simulink model "QPSK_synch_baseband"  (R2014b)
settings: Solver=VariableStepDiscrete  StartTime=0.0  StopTime=100000/fs  RelTol=1e-3
PreLoadFcn:
  | %%%%%%%%%%%%%%%%%%%%%%%%%%%%%%%%%%%%%%%%%%%%%%%%%%%%%%%%%%%%%%%%%%%%%%%%%%%
  | % check to see if Simulink library folder is missing from the MATLAB path %
  | %%%%%%%%%%%%%%%%%%%%%%%%%%%%%%%%%%%%%%%%%%%%%%%%%%%%%%%%%%%%%%%%%%%%%%%%%%%
  | if isempty(strfind(path, 'rtlsdr_book_library'))
  | 
  |     % create error window
  |     fig_error = figure(...
  |         'Name', 'Error: RTL-SDR Book Library',...
  |         'Toolbar','none',...
  |         'MenuBar','none',...
  |         'NumberTitle','off',...
  |         'Resize','off',...
  |         'WindowStyle','modal');
  |     fig_error.Position(3) = 600;
  |     fig_error.Position(4) = 150;
  |     fig_axes = axes(...
  |         'Parent',fig_error,...
  |         'Position',[0,0,1,1],...
  |         'visible','off');
  |     % error message
  |     t_title = text(.05,.8,...
  |         'MISSING DIRECTORIES',...
  |         'FontSize',11.5);
  |     t_body = text(.075,.6,...
  |         [{'Simulink cannot find the  \it{<root>}\rm / \it{rtlsdr\_book\_library}\rm  folder in the \it{MATLAB Path}\rm.'},...
  |         {'Please set the MATLAB path following the instructions given in Exercise 2.4.'}],...
  |         'FontSize',10.5);
  |     % buttons
  |     btn_path = uicontrol(...
  |         'Parent',fig_error,...
  |         'String','Set Path Now',...
  |         'FontSize',10,...
  |         'Callback', 'pathtool; close(fig_error);',...
  |         'Position', [fig_error.Position(3)/2-210, 30, 200, 30]);
  |     btn_abort = uicontrol(...
  |         'Parent',fig_error,...
  |         'String','No thanks',...
  |         'FontSize',10,...
  |         'Callback', 'close(fig_error); abort=1;',...
  |         'Position', [fig_error.Position(3)/2+10, 30, 200, 30]);
  | 
  |     % pause to allow user to interact with error box
  |     uiwait(fig_error);
  | 
  |     % abort simulation
  |     try
  |         if abort==1
  |             set_param(gcs, 'SimulationCommand', 'stop');
  |         end
  |     end
  | 
  |     % if user has set path, allow diagram to be updated
  |     if ~exist('abort','var')
  |         % create error window
  |         fig_update = figure(...
  |             'Name', 'Update Diagram',...
  |             'Toolbar','none',...
  |             'MenuBar','none',...
  |             'NumberTitle','off',...
  |             'Resize','off');
  |         fig_update.Position(3) = 400;
  |         fig_update.Position(4) = 120;
  |         fig_axes = axes(...
  |             'Parent',fig_update,...
  |             'Position',[0,0,1,1],...
  |             'visible','off');
  |         % instruction message
  |         t_body = text(.075,.7,...
  |             'Once you have set the path, update the block diagram',...
  |             'FontSize',10.5);
  |         % button
  |         btn_update = uicontrol(...
  |             'Parent',fig_update,...
  |             'String','Update Block Diagram',...
  |             'FontSize',10,...
  |             'Callback', 'set_param(gcs,''SimulationCommand'',''update''); close(gcf)',...
  |             'Position', [fig_update.Position(3)/2-100, 30, 200, 30]);
  |     end
  | 
  |     % clear error components
  |     clear('fig_error','fig_update','fig_axes','t_title','t_body','btn_path','btn_abort','btn_update','abort');
  | 
  | end
  | %%%%%%%%%%%%%%%%%%%%%%%%%%%%%%%%%%%%%%%%%%%%%%%%%%%%%%%%%%%%%%%%%%%%%%%%%%%
  | 
  | 
  | Rdata = 100e3;
  | Rsymbol = Rdata/2;
  | fs = 2.4e6;
  | MHz = fs/1e6;
  | interp = fs/Rsymbol;
  | fc = 600e3;
  | fe = 400;                   % frequency error
  | 
  | % ------- new section for synch loop design --------
  | 
  | T = 1/fs;    % sample period
  | Kp = 1;      % phase detector S-curve is linear
  | Bn = 25000;   % noise bandwidth in Hz
  | Ko = 1;      % gain of NCO (here just a direct conversion)
  | 
  | d = 0.707;  % damping ratio
  | 
  | % calculate the loop filter coefficients
  | K1 = (4*d*Bn*T)/(Ko*Kp*(d+1/(4*d)));
  | K2 = (4*(Bn*T)^2)/(Ko*Kp*(d+1/4*d)^2);
undefined symbols (not defined in the file): startfcn_constellation, startfcn_time_scope
libraries: commfilt2 x4, commrandsrc2 x1, rtlsdr_book_library x1, commdigbbndpm3 x1
CloseFcn:
  | closefcn_model;
Description:
  | Software, Simulation Examples and Design Exercises Licence Agreement
  | 
  | This license agreement refers to the simulation examples, design exercises and files,
  | and associated software MATLAB and Simulink resources that accompany the book:
  | 
  |      Title: Software Defined Radio using MATLAB & Simulink and the RTL-SDR
  |      Published by Strathclyde Academic Media, 2015
  |      Authored by Robert W. Stewart, Kenneth W. Barlee, Dale S.W. Atkinson,
  |      and Louise H. Crockett
  | 
  | and made available as a download from, www.desktopSDR.com or variously acquired
  | by other means such as via USB storage, cloud storage, disk or any other electronic
  | or optical or magnetic storage mechanism. These files and associated software may
  | be used subject to the terms of agreement of the conditions below:
  | 
  |     Copyright © 2015 Robert W. Stewart, Kenneth W. Barlee, Dale S.W. Atkinson,
  |     and Louise H. Crockett
  |     All rights reserved.
  | 
  | Redistribution and use in source and binary forms, with or without modification, are
  | permitted provided that the following conditions are met:
  | 
  |    1.  Redistributions of source code must retain the above copyright notice, this list of
  |         conditions and the following disclaimer.
  | 
  |    2.  Redistributions in binary form must reproduce the above copyright notice, this
  |         list of conditions and the following disclaimer in the documentation and/or other
  |         materials provided with the distribution.
  | 
  |    3.  Neither the name of the copyright holder nor the names of its contributors may
  |         be used to endorse or promote products derived from this software without
  |         specific prior written permission.
  | 
  |    4.  In all cases, the software is, and all modifications and derivatives of the
  |         software shall be, licensed to you solely for use in conjunction with The
  |         MathWorks, Inc. products and service offerings.
  | 
  | THIS SOFTWARE IS PROVIDED BY THE COPYRIGHT HOLDERS AND CONTRIBUTORS
  | "AS IS" AND ANY EXPRESS OR IMPLIED WARRANTIES, INCLUDING, BUT NOT LIMITED
  | TO, THE IMPLIED WARRANTIES OF MERCHANTABILITY AND FITNESS FOR A
  | PARTICULAR PURPOSE ARE DISCLAIMED. IN NO EVENT SHALL THE COPYRIGHT
  | HOLDER OR CONTRIBUTORS BE LIABLE FOR ANY DIRECT, INDIRECT, INCIDENTAL,
  | SPECIAL, EXEMPLARY, OR CONSEQUENTIAL DAMAGES (INCLUDING, BUT NOT
  | LIMITED TO, PROCUREMENT OF SUBSTITUTE GOODS OR SERVICES; LOSS OF USE,
  | DATA, OR PROFITS; OR BUSINESS INTERRUPTION) HOWEVER CAUSED AND ON ANY
  | THEORY OF LIABILITY, WHETHER IN CONTRACT, STRICT LIABILITY, OR TORT
  | (INCLUDING NEGLIGENCE OR OTHERWISE) ARISING IN ANY WAY OUT OF THE USE
  | OF THIS SOFTWARE, EVEN IF ADVISED OF THE POSSIBILITY OF SUCH DAMAGE.
  | 
  | 
  | Audio Tracks used in Simulations Examples and Design Exercises
  | 
  | The music and vocal files used within the Examples files and software within the book
  | were variously written, arranged, performed, recorded and produced by Garrey Rice,
  | Adam Struth, Jamie Struth, Iain Thistlethwaite and also Marshall Craigmyle who
  | collectively, and individually where appropriate, assert and retain all of their copyright,
  | performance and artistic rights. Permission to use and reproduce this music is
  | granted for all purposes associated with MATLAB and Simulink software and the
  | simulation examples and design exercises files that accompany this book. Requests to
  | use the music for any other purpose should be directed to: info@desktopSDR.com.
  | For information on music track names, full credits, and links to the musicians please
  | refer to www.desktopSDR.com/more/audio.
settings Model: Creator=desktopSDR Team  LastModifiedBy=desktopSDR Team
settings DataIOCC: LimitDataPoints=off  SaveOutput=off  SignalLogging=off  SaveTime=off
settings DebuggingCC: UnderspecifiedInitializationDetection=Classic  MergeDetectMultiDrivingBlocksExec=none

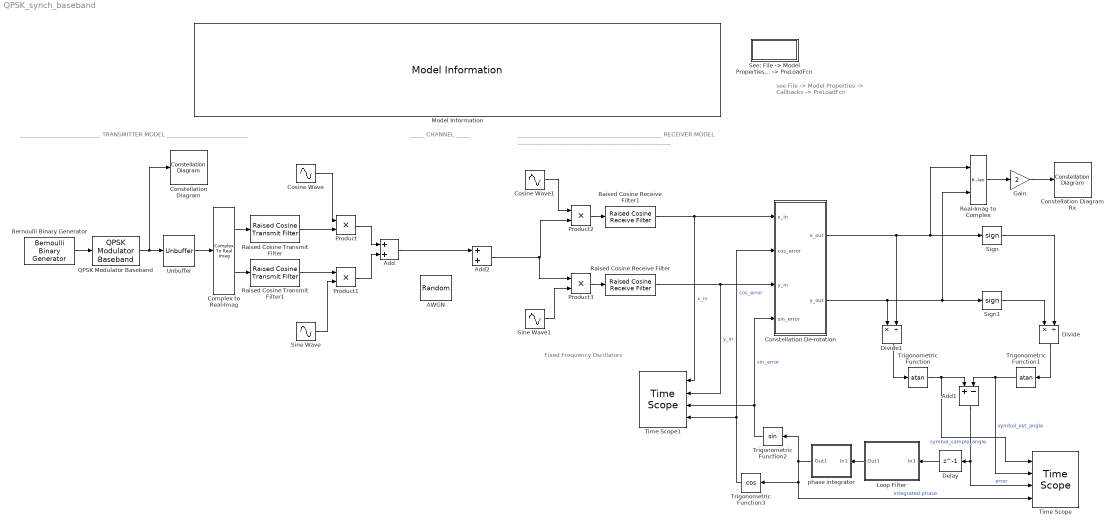
== system QPSK_synch_baseband ==
  note: Fixed Frequency
      | Oscillators
  note: ___________________________ TRANSMITTER MODEL ___________________________
  note: _____ CHANNEL _____
  note: ________________________________________________ RECEIVER MODEL ___________________________________________________
  note: see File -> Model Properties
      | -> Callbacks -> PreLoadFcn
  AWGN : RandomNumber  Variance=0.001  Seed=555  SampleTime=1/fs
  Add : Sum
  Add1 : Sum  Inputs=+-
  Add2 : Sum
  Bernoulli Binary Generator : commrandsrc2/Bernoulli Binary Generator  P=0.5  seed=61  Ts=1/Rdata  frameBased=on  sampPerFrame=2  orient=off  outDataType=double
  Complex to Real-Imag : ComplexToRealImag
  Constellation De-rotation : Subsystem
  Constellation Diagram : ConstellationDiagram  StartFcn=startfcn_constellation;
  Constellation Diagram Rx : ConstellationDiagram  StartFcn=startfcn_constellation;
  Cosine Wave : Sin  Frequency=(fc+fe)*2*pi  Phase=pi/2  SampleTime=1/fs
  Cosine Wave1 : Sin  Frequency=fc*2*pi  Phase=pi/2  SampleTime=1/fs
  Delay : Delay  DelayLength=1
  Divide : Product  Inputs=*/
  Divide1 : Product  Inputs=*/
  Gain : Gain  Gain=2
  Loop Filter : Subsystem
  Model Information : rtlsdr_book_library/Additional Tools/Model Information/Model Information
  Product{,1..3} (4 alike) : Product
  QPSK Modulator Baseband : commdigbbndpm3/QPSK Modulator Baseband  InType=Bit  Enc=Gray  Ph=pi/4  outDtype=double  outWordLen=16  outUDDataType=sfix(16)  outFracLenMode=Best precision  outFracLen=15
  Raised Cosine Receive Filter : commfilt2/Raised Cosine Receive Filter  filtType=Square root  N=interp  filtSpan=8  currentFiltSpan=8  D=(8)/2  R=0.25  sampMode=Mute  saveAsFlag=0  rateMode=Downsampling  downFactor=interp  downOffset=0  framing=Allow multirate processing  checkGain=Normalized  filterGain=1  checkCoeff=off  variableName=rcRxFilt  launchFVT=on  roundingMode=Floor  overflowMode=off
  Raised Cosine Receive Filter1 : commfilt2/Raised Cosine Receive Filter  filtType=Square root  N=interp  filtSpan=8  currentFiltSpan=8  D=(8)/2  R=0.25  sampMode=Mute  saveAsFlag=0  rateMode=Downsampling  downFactor=interp  downOffset=0  framing=Allow multirate processing  checkGain=Normalized  filterGain=1  checkCoeff=off  variableName=rcRxFilt1  launchFVT=on  roundingMode=Floor  overflowMode=off
  Raised Cosine Transmit Filter : commfilt2/Raised Cosine Transmit Filter  filtType=Square root  filtSpan=8  currentFiltSpan=8  D=(8)/2  R=0.25  sampMode=Mute  saveAsFlag=0  N=interp  framing=Allow multirate processing  checkGain=Normalized  filterGain=1  checkCoeff=off  variableName=rcTxFilt  launchFVT=on  roundingMode=Floor  overflowMode=off
  Raised Cosine Transmit Filter1 : commfilt2/Raised Cosine Transmit Filter  filtType=Square root  filtSpan=8  currentFiltSpan=8  D=(8)/2  R=0.25  sampMode=Mute  saveAsFlag=0  N=interp  framing=Allow multirate processing  checkGain=Normalized  filterGain=1  checkCoeff=off  variableName=rcTxFilt1  launchFVT=on  roundingMode=Floor  overflowMode=off
  Real-Imag to Complex : RealImagToComplex
  "See: File -> Model Properties -> Callbacks -> PreLoadFcn " : Subsystem
      mask Display:
      | MHz = evalin('base', 'MHz');
      | fprintf(['fs = ',num2str(MHz),' MHz']);
  Sign : Signum
  Sign1 : Signum
  Sine Wave : Sin  Frequency=(fc+fe)*2*pi  SampleTime=1/fs
  Sine Wave1 : Sin  Frequency=fc*2*pi  SampleTime=1/fs
  Time Scope : TimeScope  StartFcn=startfcn_time_scope;  DefaultConfigurationName=spbscopes.TimeScopeBlockCfg  NumInputPorts=4
  Time Scope1 : TimeScope  StartFcn=startfcn_time_scope;  DefaultConfigurationName=spbscopes.TimeScopeBlockCfg  NumInputPorts=4
  Trigonometric Function : Trigonometry  Operator=atan  OutputSignalType=real
  Trigonometric Function1 : Trigonometry  Operator=atan  OutputSignalType=real
  Trigonometric Function2 : Trigonometry
  Trigonometric Function3 : Trigonometry  Operator=cos
  Unbuffer : Unbuffer  SampleBasedProcessing=Same as frame based
  phase integrator : Subsystem
  wires:
  Bernoulli Binary Generator/1 -> QPSK Modulator Baseband/1
  QPSK Modulator Baseband/1 -> Unbuffer/1, Constellation Diagram/1
  Complex to Real-Imag/1 -> Raised Cosine Transmit Filter/1
  Complex to Real-Imag/2 -> Raised Cosine Transmit Filter1/1
  Raised Cosine Transmit Filter/1 -> Product/2
  Raised Cosine Transmit Filter1/1 -> Product1/1
  Sine Wave/1 -> Product1/2
  Unbuffer/1 -> Complex to Real-Imag/1
  Cosine Wave/1 -> Product/1
  Product2/1 -> Raised Cosine Receive Filter1/1
  Product3/1 -> Raised Cosine Receive Filter/1
  Real-Imag to Complex/1 -> Gain/1
  Gain/1 -> Constellation Diagram Rx/1
  Product/1 -> Add/1
  Product1/1 -> Add/2
  Sign/1 -> Divide/2
  Sign1/1 -> Divide/1
  Trigonometric Function/1 -> Add1/1, Time Scope/1  "symbol_sample_angle"
  Trigonometric Function1/1 -> Time Scope/2, Add1/2  "symbol_est_angle"
  Loop Filter/1(Out1) -> phase integrator/1(In1)
  Cosine Wave1/1 -> Product2/1
  Trigonometric Function2/1 -> Time Scope1/3, Constellation De-rotation/4(sin_error)  "sin_error"
  Constellation De-rotation/1(x_out) -> Sign/1, Real-Imag to Complex/1, Divide1/2
  Constellation De-rotation/2(y_out) -> Sign1/1, Real-Imag to Complex/2, Divide1/1
  Raised Cosine Receive Filter1/1 -> Time Scope1/1, Constellation De-rotation/1(x_in)  "x_in"
  Raised Cosine Receive Filter/1 -> Time Scope1/2, Constellation De-rotation/3(y_in)  "y_in"
  Trigonometric Function3/1 -> Time Scope1/4, Constellation De-rotation/2(cos_error)  "cos_error"
  Add/1 -> Add2/1
  Add2/1 -> Product3/1, Product2/2
  Divide/1 -> Trigonometric Function1/1
  Divide1/1 -> Trigonometric Function/1
  Delay/1 -> Loop Filter/1(In1)
  Sine Wave1/1 -> Product3/2
  Add1/1 -> Time Scope/3, Delay/1  "error"
  phase integrator/1(Out1) -> Trigonometric Function2/1, Time Scope/4, Trigonometric Function3/1  "integrated phase"

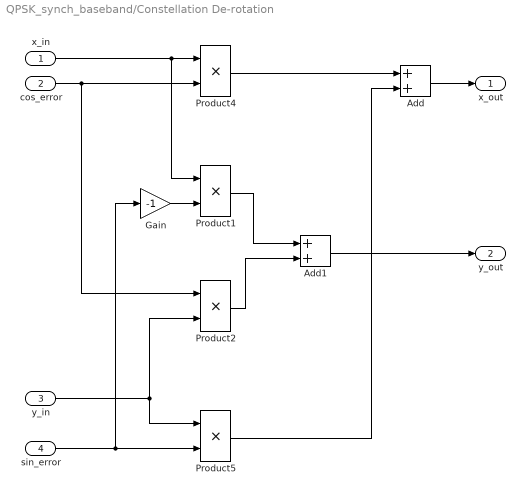
== system QPSK_synch_baseband/Constellation De-rotation ==
  x_in : Inport
  cos_error : Inport  Port=2
  y_in : Inport  Port=3
  sin_error : Inport  Port=4
  Add : Sum
  Add1 : Sum
  Gain : Gain  Gain=-1
  Product{1..2,4..5} (4 alike) : Product
  x_out : Outport
  y_out : Outport  Port=2
  wires:
  Product4/1 -> Add/1
  y_in/1 -> Product2/2, Product5/1
  sin_error/1 -> Gain/1, Product5/2
  x_in/1 -> Product1/1, Product4/1
  Product5/1 -> Add/2
  cos_error/1 -> Product2/1, Product4/2
  Add/1 -> x_out/1
  Gain/1 -> Product1/2
  Product2/1 -> Add1/2
  Product1/1 -> Add1/1
  Add1/1 -> y_out/1

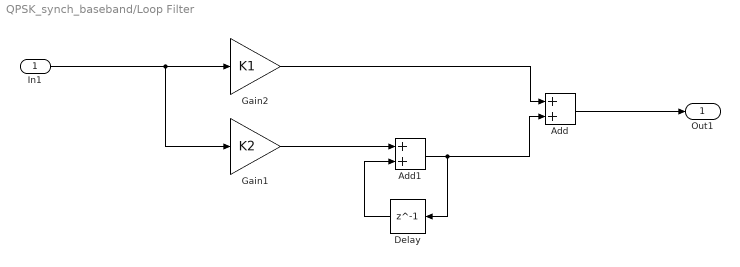
== system QPSK_synch_baseband/Loop Filter ==
  In1 : Inport
  Add : Sum
  Add1 : Sum
  Delay : Delay  DelayLength=1
  Gain1 : Gain  Gain=K2
  Gain2 : Gain  Gain=K1
  Out1 : Outport
  wires:
  Add/1 -> Out1/1
  Gain2/1 -> Add/1
  Delay/1 -> Add1/2
  Add1/1 -> Delay/1, Add/2
  Gain1/1 -> Add1/1
  In1/1 -> Gain1/1, Gain2/1

== system QPSK_synch_baseband/See: File -> Model Properties -> Callbacks -> PreLoadFcn  ==

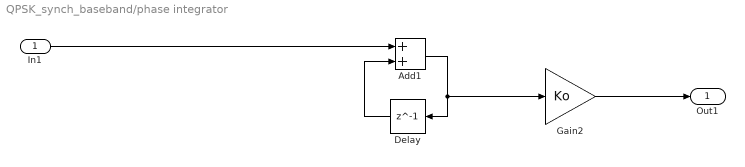
== system QPSK_synch_baseband/phase integrator ==
  In1 : Inport
  Add1 : Sum
  Delay : Delay  DelayLength=1
  Gain2 : Gain  Gain=Ko
  Out1 : Outport
  wires:
  In1/1 -> Add1/1
  Add1/1 -> Gain2/1, Delay/1
  Delay/1 -> Add1/2
  Gain2/1 -> Out1/1
